simulink model "ejemplo_ruido"  (R2021a)
settings: Solver=ode45  StartTime=0.0  StopTime=10.0  RelTol=1e-3  EnableMultiTasking=on
values from neighbouring files (symbols this model uses):
  C = 3  6  9 12 15    [tp1.m]    (also in tp3.m = FaC(F))
undefined symbols (not defined in the file or in its folder): none, Rec, SDTV, videoinput
libraries: visionconversions x1, imaqlib x1, visionanalysis x1
settings Model: Creator=eae  LastModifiedBy=ZeK005
settings SolverCC: AlgebraicLoopSolver=TrustRegion
settings DataIOCC: LimitDataPoints=on  SaveFormat=Array  ReturnWorkspaceOutputs=off
settings OptimizationCC: LifeSpan=inf
settings DebuggingCC: UnderspecifiedInitializationDetection=Classic  MergeDetectMultiDrivingBlocksExec=none  SolverPrmCheckMsg=warning  StateNameClashWarn=warning  SFUnexpectedBacktrackingDiag=warning  SFNoUnconditionalDefaultTransitionDiag=warning  SFExecutionAtInitializationDiag=none  SFMachineParentedDataDiag=warning  ArithmeticOperatorsInVariantConditions=warning
settings HardwareCC: ProdBitPerPointer=32  ProdBitPerSizeT=32  ProdBitPerPtrDiffT=32  ProdLargestAtomicFloat=None  ProdIntDivRoundTo=Undefined  ProdEndianess=Unspecified  ProdWordSize=32  ProdHWDeviceType=32-bit Generic
settings ModelReferenceCC: PropagateSignalLabelsOutOfModel=off
settings SFSimCC: SimUseLocalCustomCode=off  CustomCodeUndefinedFunction=UseInterfaceOnly
settings RTWCC: RTWUseLocalCustomCode=off
settings CodeAppCC: StateflowObjectComments=on
settings GRTTargetCC: TargetLangStandard=C89/C90 (ANSI)
settings ConfigComp: CovMetricSettings=dw  CovSaveCumulativeToWorkspaceVar=on  CovSaveSingleToWorkspaceVar=on  CovExternalEMLEnable=off

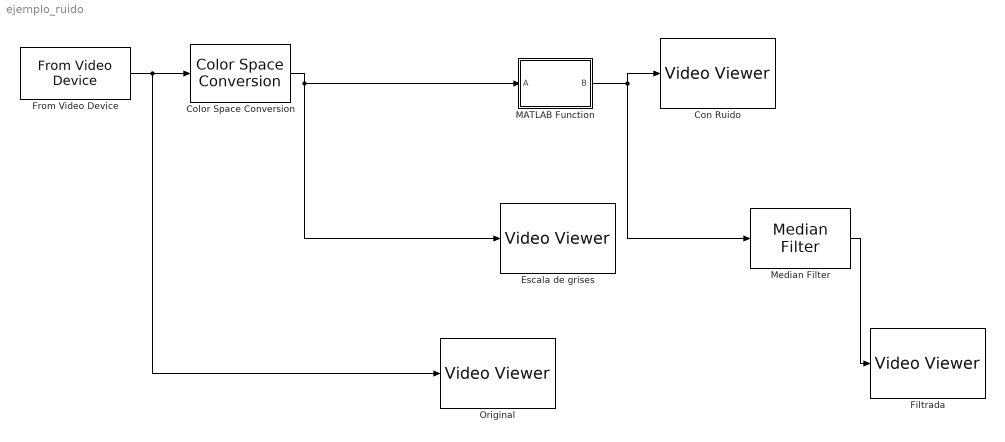
== system ejemplo_ruido ==
  Color Space Conversion : visionconversions/Color Space  Conversion  conversion=Obsolete  conversionActive=R'G'B' to intensity  wp_str=D65  rec=Rec. 601 (SDTV)  sys=1125/60/2:1  imagePorts=One multidimensional signal
  Con Ruido : VideoViewer  FigPos=[871 449 410 300]
  Escala de grises : VideoViewer  FigPos=[90 899 410 300]
  Filtrada : VideoViewer  FigPos=[1369 433 410 300]
  From Video Device : imaqlib/From Video Device  DeviceMenu=winvideo 1 (HD Pro Webcam C920)  Device=winvideo 1 (HD Pro Webcam C920)  ObjConstructor=videoinput('winvideo', 1)  VideoFormatMenu=MJPG_640x480  VideoFormat=MJPG_640x480  VideoSource=input1  ROIPosition=[0 0 480 640]  EnableHWTrigger=off  TriggerConfiguration=none/none  SampleTime=1/30  OutputPortsMode=One multidimensional signal  DataType=single  CanDoHWTrigger=no  ReturnedColorSpace=rgb  BlockHandle=1965.0002  ROIWidth=640  ROIHeight=480  ROIColumn=0  ROIRow=0  EngXMLPath=C:\Program Files\Polyspace\R2021a\toolbox\imaq\imaq\private  DevXMLPath=C:\ProgramData\MATLAB\SupportPackages\R2021a\toolbox\imaq\supportpackages\genericvideo\adaptor\win64  EngLibPath=C:\Program Files\Polyspace\R2021a\toolbox\imaq\imaqblks\imaqmex\win64  ColorSpace=rgb  BayerSensorAlignment=grbg  ImaqMode=off
  MATLAB Function : MATLAB Function  TreatAsAtomicUnit=on
  Median Filter : visionanalysis/Median Filter  nghbood=[3 3]  outSize=Same as input port I  padType=Constant  padSrc=Specify via dialog  padVal=0  roundingMode=Floor  overflowMode=off
      settings: SourceProductBaseCode=VP
  Original : VideoViewer  FigPos=[50 416 410 300]
  wires:
  Color Space Conversion/1 -> Escala de grises/1, MATLAB Function/1(A)
  From Video Device/1 -> Original/1, Color Space Conversion/1
  MATLAB Function/1(B) -> Con Ruido/1, Median Filter/1
  Median Filter/1 -> Filtrada/1

== matlab function ejemplo_ruido/MATLAB Function ==
  data: A input; B output
function B = ruidopro(A)
%ruido
B=A;
%se obtiene el tamaño de la imagen
[m n]=size(A);
%Se distorcionan 300 puntos de la imagen con ruido sal
for v=1:10000
    % Se obtiene la posicion del pixel a distorsionar    
    x=round((m-1)*rand);
    y=round((n-1)*rand);
    % Se protege si el valor obtenido es cero
    if(x==0)
        x=1;
    end
    % Se protege si el valor obtenido es cero
    if(y==0)
        y=1;
    end
    %se distorsiona el pixel
    B(x,y)=1;
end
% Se distorsionan 300 puntos de la imagen con ruido pimienta 
for v=1:10000
    x=round((m-1)*rand);
    y=round((n-1)*rand);
    if(x==0)
        x=1;
    end
    if(y==0)
        y=1;
    end
    B(x,y)=0;
end
